simulink model "DC_SERIES_WOUND"  (R2021a)
settings: Solver=VariableStepAuto  StartTime=0.0  StopTime=10.0  RelTol=1e-3
values from neighbouring files (symbols this model uses):
  A = 0.1    [Kibble_Simu_4.m]    (also in Kibble_Simulation_code2.m; LQG.m = [1.1269   -0.4940    0.1129; LQG_TEST2.m = [0 1 0 0; LQR.m = [0 1 0 0)
  N = 0    [LQG.m]    (also in LQG_TEST2.m; LQR.m = [0; 0; 0;0])
libraries: spsDCVoltageSourceLib x2, spsDCMachineLib x1, spsVoltageMeasurementLib x1, spspowerguiLib x1
settings Model: Creator=HP  LastModifiedBy=HP
settings SolverCC: ZeroCrossAlgorithm=Adaptive
settings DebuggingCC: IgnoredZcDiagnostic=none

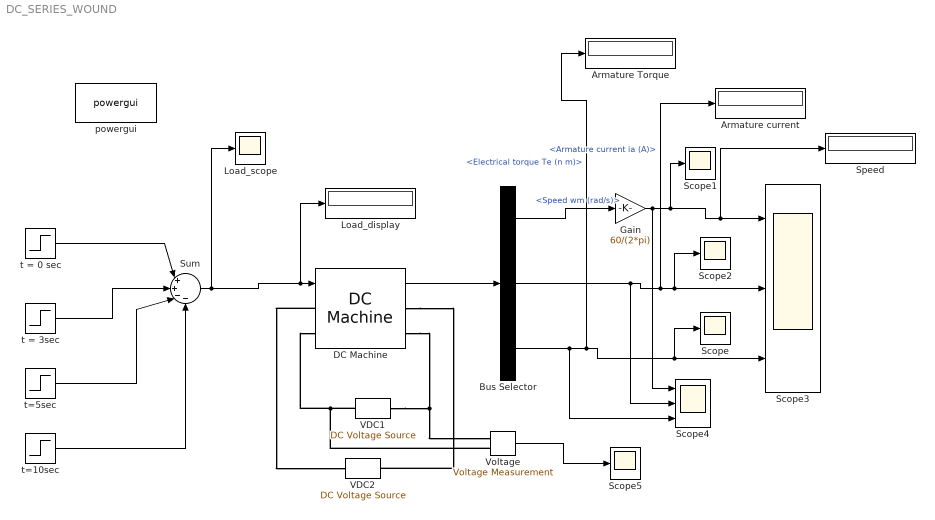
== system DC_SERIES_WOUND ==
  Armature Torque : Display
  Armature current : Display
  Bus Selector : BusSelector  OutputSignals=Speed wm (rad/s),Armature current ia (A),Electrical torque Te (n m)
  DC Machine : spsDCMachineLib/DC Machine  PresetModel=01: 5HP 240V 1750RPM Field:300V  MechanicalLoad=Torque TL  FieldType=Wound  ShowDetailedParameters=on  MeasurementBus=off  RLa=[2.581 0.028]  RLf=[281.2 156]  Laf=0.9483  MachineConstant=Torque constant (N.m/A)  Ke=1.8  Kt=1.8  J=0.02215  Bm=0.002953  Tf=0.5161  w0=1  Ifinit=0.00510100335041874  TsPowergui=0  TsBlock=-1
  Gain : Gain  Gain=60/(2*pi)
  Load_display : Display
  Load_scope : Scope
  Scope{,1..2,5} (4 alike) : Scope
  Scope3 : Scope  NumInputPorts=3
  Scope4 : Scope  NumInputPorts=3
  Speed : Display
  Sum : Sum  Inputs=|++--
  VDC1 : spsDCVoltageSourceLib/DC Voltage Source  Amplitude=300  Measurements=None
  VDC2 : spsDCVoltageSourceLib/DC Voltage Source  Amplitude=240  Measurements=None
  Voltage : spsVoltageMeasurementLib/Voltage Measurement  PhasorSimulation=off  OutputType=Complex  PSBequivalent=0
  powergui : spspowerguiLib/powergui  Priority=1  SimulationMode=Continuous  SampleTime=50e-6  frequency=60  Iterations=50  frequencyindice=0  Pbase=100e6  ErrMax=1e-4  UnitsV=kV  UnitsW=MW  buscounter=0  FunctionMessages=off  echomessages=off  EnableUseOfTLC=off  CurrentSourceSwitches=off  DisableSnubberDevices=off  DisableRonSwitches=off  DisableVfSwitches=off  DisplayEquations=off  AutomaticDiscreteSolvers=off  SolverType=Tustin/Backward Euler (TBE)  Interpol=off  ExternalGateDelay=off  methode=off  Ts=100  x0status=blocks  SPID=on  SwTol=0  HookPort=off  NonlinearTolerance=1e-4  nMaxIteration=100  ContinueOnMaxIteration=off  RestoreLinks=warning  ResistiveCurrentMeasurement=off  Frange=[0:2:500]  Ylog=off  Xlog=on  ShowGrid=off  save=off  variable=ZData  structure=0  ZoomFFT=off  StartTime=0.0  cycles=1  DisplayStyle=1  fundamental=60  FreqAxis=off  MaxFrequency=1000  frequencyindicesteady=1  RmsSteady=1  display=off
  t = 0 sec : Step  Time=0  After=0  SampleTime=0
  "t = 3sec " : Step  Time=3  After=20.36  SampleTime=0
  t=10sec : Step  Time=10  After=5.09  SampleTime=0
  t=5sec : Step  Time=5  After=10.18  SampleTime=0
  wires:
  DC Machine/1 -> Bus Selector/1
  Bus Selector/1 -> Gain/1  "<Speed wm (rad/s)>"
  Bus Selector/2 -> Scope4/2, Armature current/1, Scope2/1, Scope3/2  "<Armature current ia (A)>"
  Bus Selector/3 -> Scope4/3, Armature Torque/1, Scope/1, Scope3/3  "<Electrical torque Te (n m)>"
  Gain/1 -> Scope4/1, Scope1/1, Speed/1, Scope3/1
  Sum/1 -> Load_scope/1, Load_display/1, DC Machine/1
  t = 0 sec/1 -> Sum/1
  "t = 3sec "/1 -> Sum/2
  t=5sec/1 -> Sum/3
  t=10sec/1 -> Sum/4
  Voltage/1 -> Scope5/1
  connections:
  Voltage/LConn2 -- DC Machine/LConn2 -- VDC1/LConn1
  DC Machine/RConn2 -- VDC1/RConn1 -- Voltage/LConn1
  DC Machine/LConn1 -- VDC2/LConn1
  DC Machine/RConn1 -- VDC2/RConn1
